simulink model "SimulinkProjet"  (R2016b)
settings: Solver=ode3  StartTime=0.0  StopTime=inf  FixedStep=Te  RelTol=1e-3
values from neighbouring files (symbols this model uses):
  Te = 0.001    [MatlabProjet.m]
libraries: xpcnilib x2, simulink x2, simulink_extras x1
settings Model: SimulationMode=external  Creator=luhernan  LastModifiedBy=USUARIO
settings SolverCC: EnableConcurrentExecution=on
settings DataIOCC: SaveFormat=StructureWithTime
settings OptimizationCC: BlockReduction=off  OptimizeBlockIOStorage=off  BufferReuse=off  GlobalBufferReuse=off  ExpressionFolding=off  LocalBlockOutputs=off  LifeSpan=inf
settings DebuggingCC: SFUnexpectedBacktrackingDiag=warning  SFNoUnconditionalDefaultTransitionDiag=warning  SFExecutionAtInitializationDiag=none
settings HardwareCC: ProdBitPerPointer=32  ProdBitPerSizeT=32  ProdBitPerPtrDiffT=32  ProdLargestAtomicFloat=None  ProdWordSize=32  ProdLongLongMode=on  ProdHWDeviceType=Generic->32-bit x86 compatible
settings RTWCC: SystemTargetFile=slrt.tlc  TemplateMakefile=slrt_default_tmf  Description=Simulink Real-Time  RTWCompilerOptimization=on
settings ConfigComp: CovMetricSettings=dw  CovHtmlReporting=on  CovSaveCumulativeToWorkspaceVar=on  CovSaveSingleToWorkspaceVar=on  CovExternalEMLEnable=off

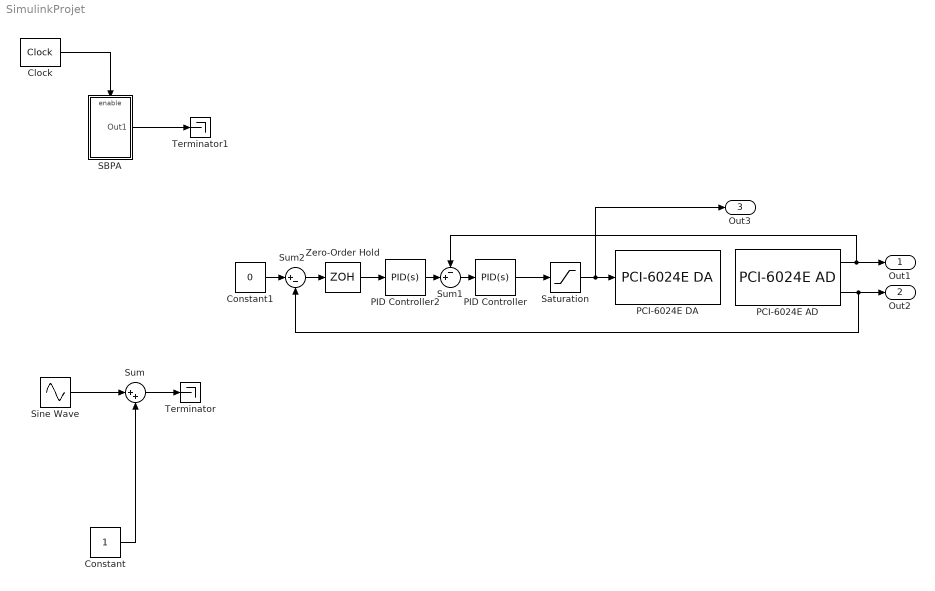
== system SimulinkProjet ==
  Clock : simulink_extras/Flip Flops/Clock  period=PHorloge
  Constant : Constant
  Constant1 : Constant  Value=0
  PCI-6024E AD : xpcnilib/A//D/E Series/PCI-6024E AD  channel=[1,2]  range=[-10]  coupling=[0]  sampletime=Te  slot=-1
  PCI-6024E DA : xpcnilib/D//A/E Series/PCI-6024E DA  channel=[1]  reset=[1]  initValue=[0]  sampletime=Te  slot=-1
  PID Controller : simulink/Continuous/PID Controller  Controller=PID  TimeDomain=Continuous-time  SampleTime=-1  IntegratorMethod=Forward Euler  FilterMethod=Forward Euler  Form=Parallel  UseFilter=on  ControllerParametersSource=internal  P=-2.5  I=-5  D=0  N=100  InitialConditionSource=internal  InitialConditionForIntegrator=0  InitialConditionForFilter=0  ExternalReset=none  LimitOutput=off  UpperSaturationLimit=inf  LowerSaturationLimit=-inf  LinearizeAsGain=on  AntiWindupMode=none  Kb=1  TrackingMode=off  Kt=1  PParamMin=[]  PParamMax=[]  IParamMin=[]  IParamMax=[]  DParamMin=[]  DParamMax=[]  NParamMin=[]  NParamMax=[]  KbParamMin=[]  KbParamMax=[]  KtParamMin=[]  KtParamMax=[]  POutMin=[]  POutMax=[]  IOutMin=[]  IOutMax=[]  DOutMin=[]  DOutMax=[]  NOutMin=[]  NOutMax=[]  KbOutMin=[]  KbOutMax=[]  KtOutMin=[]  KtOutMax=[]  IntegratorOutMin=[]  IntegratorOutMax=[]  FilterOutMin=[]  FilterOutMax=[]  SumOutMin=[]  SumOutMax=[]  SumI1OutMin=[]  SumI1OutMax=[]  SumI2OutMin=[]  SumI2OutMax=[]  SumI3OutMin=[]  SumI3OutMax=[]  SumDOutMin=[]  SumDOutMax=[]  SaturationOutMin=[]  SaturationOutMax=[]  IntegratorContinuousStateAttributes=''  IntegratorStateMustResolveToSignalObject=off  IntegratorRTWStateStorageClass=Auto  FilterContinuousStateAttributes=''  FilterStateMustResolveToSignalObject=off  FilterRTWStateStorageClass=Auto  DifferentiatorICPrevScaledInput=0  DifferentiatorOutMin=[]  DifferentiatorOutMax=[]
  PID Controller2 : simulink/Continuous/PID Controller  Controller=PID  TimeDomain=Continuous-time  SampleTime=-1  IntegratorMethod=Forward Euler  FilterMethod=Forward Euler  Form=Parallel  UseFilter=on  ControllerParametersSource=internal  P=0.8514  I=0.05070  D=0.8008  N=5  InitialConditionSource=internal  InitialConditionForIntegrator=0  InitialConditionForFilter=0  ExternalReset=none  LimitOutput=off  UpperSaturationLimit=inf  LowerSaturationLimit=-inf  LinearizeAsGain=on  AntiWindupMode=none  Kb=1  TrackingMode=off  Kt=1  PParamMin=[]  PParamMax=[]  IParamMin=[]  IParamMax=[]  DParamMin=[]  DParamMax=[]  NParamMin=[]  NParamMax=[]  KbParamMin=[]  KbParamMax=[]  KtParamMin=[]  KtParamMax=[]  POutMin=[]  POutMax=[]  IOutMin=[]  IOutMax=[]  DOutMin=[]  DOutMax=[]  NOutMin=[]  NOutMax=[]  KbOutMin=[]  KbOutMax=[]  KtOutMin=[]  KtOutMax=[]  IntegratorOutMin=[]  IntegratorOutMax=[]  FilterOutMin=[]  FilterOutMax=[]  SumOutMin=[]  SumOutMax=[]  SumI1OutMin=[]  SumI1OutMax=[]  SumI2OutMin=[]  SumI2OutMax=[]  SumI3OutMin=[]  SumI3OutMax=[]  SumDOutMin=[]  SumDOutMax=[]  SaturationOutMin=[]  SaturationOutMax=[]  IntegratorContinuousStateAttributes=''  IntegratorStateMustResolveToSignalObject=off  IntegratorRTWStateStorageClass=Auto  FilterContinuousStateAttributes=''  FilterStateMustResolveToSignalObject=off  FilterRTWStateStorageClass=Auto  DifferentiatorICPrevScaledInput=0  DifferentiatorOutMin=[]  DifferentiatorOutMax=[]
  SBPA : Subsystem  mask{A=14, Offset=-6}
      mask prompts: A "gain"
  Saturation : Saturate  UpperLimit=10  LowerLimit=-10
  Sine Wave : Sin  Amplitude=9  Frequency=6*pi  SampleTime=Te
  Sum : Sum  Inputs=|++
  Sum1 : Sum  Inputs=-+|
  Sum2 : Sum  Inputs=|+-
  Terminator : Terminator
  Terminator1 : Terminator
  Zero-Order Hold : ZeroOrderHold  SampleTime=Te
  Out1 : Outport
  Out2 : Outport  Port=2
  Out3 : Outport  Port=3
  wires:
  Constant/1 -> Sum/2
  Sine Wave/1 -> Sum/1
  Sum/1 -> Terminator/1
  Clock/1 -> SBPA/Enable
  SBPA/1(Out1) -> Terminator1/1
  PCI-6024E AD/1 -> Sum1/1, Out1/1
  PID Controller/1 -> Saturation/1
  PCI-6024E AD/2 -> Sum2/2, Out2/1
  Constant1/1 -> Sum2/1
  Sum2/1 -> Zero-Order Hold/1
  PID Controller2/1 -> Sum1/2
  Sum1/1 -> PID Controller/1
  Zero-Order Hold/1 -> PID Controller2/1
  Saturation/1 -> Out3/1, PCI-6024E DA/1

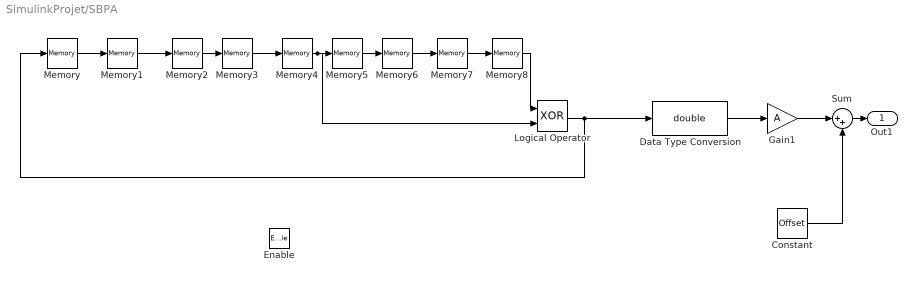
== system SimulinkProjet/SBPA ==
  Enable : EnablePort
  Constant : Constant  Value=Offset
  Data Type Conversion : DataTypeConversion  OutMin=[0]  OutMax=[5]  OutDataTypeStr=double
  Gain1 : Gain  Gain=A
  Logical Operator : Logic  Operator=XOR  AllPortsSameDT=off  OutDataTypeStr=boolean
  Memory : Memory  X0=1  InheritSampleTime=on
  Memory{1..8} (8 alike) : Memory  InheritSampleTime=on
  Sum : Sum  Inputs=|++
  Out1 : Outport
  wires:
  Logical Operator/1 -> Memory/1, Data Type Conversion/1
  Memory1/1 -> Memory2/1
  Memory/1 -> Memory1/1
  Memory2/1 -> Memory3/1
  Data Type Conversion/1 -> Gain1/1
  Memory3/1 -> Memory4/1
  Memory4/1 -> Logical Operator/2, Memory5/1
  Memory5/1 -> Memory6/1
  Memory6/1 -> Memory7/1
  Memory7/1 -> Memory8/1
  Memory8/1 -> Logical Operator/1
  Constant/1 -> Sum/2
  Gain1/1 -> Sum/1
  Sum/1 -> Out1/1
